simulink model "pv_model"  (R2024b)
settings: Solver=VariableStepAuto  StartTime=0.0  StopTime=1.5  RelTol=1e-3
libraries: simulink x1
settings Model: Creator=vasudha  LastModifiedBy=vasudha
settings DebuggingCC: AlgebraicLoopMsg=none

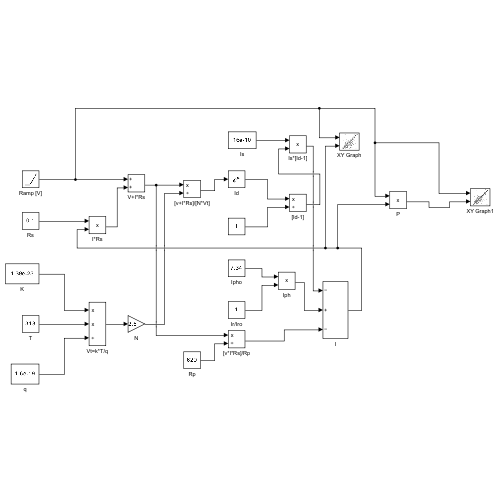
[thumbnail: Simulink's stored preview of the top-level diagram]
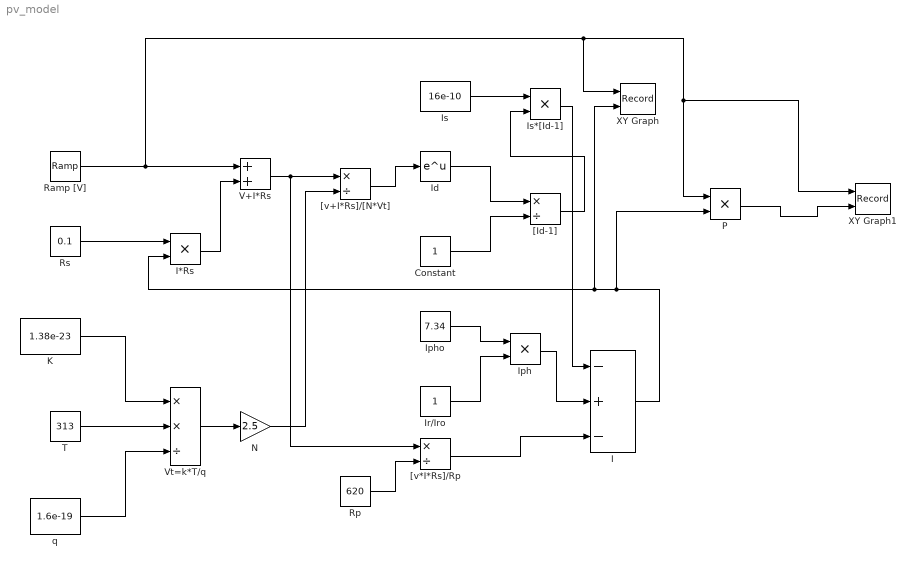
== system pv_model ==
  Constant : Constant
  I : Sum  Inputs=-+-
  I*Rs : Product
  Id : Math
  Iph : Product
  Ipho : Constant  Value=7.34
  Ir/Iro : Constant
  Is : Constant  Value=16e-10
  Is*[Id-1] : Product
  K : Constant  Value=1.38e-23
  N : Gain  Gain=2.5
  P : Product
  Ramp [V] : simulink/Sources/Ramp  slope=1  start=0  InitialOutput=0
  Rp : Constant  Value=620
  Rs : Constant  Value=0.1
  T : Constant  Value=313
  V+I*Rs : Sum
  Vt=k*T/q : Product  Inputs=**/
  XY Graph : Record  FileSettingsInternal="{\"entries\":[{\"content\":{\"excelSettings\":{\"content\":{},\"type\":\"Streamout.ExcelSettings\"}},\"type\":\"Streamout.FileSettingStorage\",\"uuid\":\"\"}],\"packageUris\":[\"http:\\/\\/schema.mathworks.com\\/mf0\\/streamout_blocks\\/R2020a\"],\"version\":\"1.0\"}"  Layout=[1 1]  SignalsInternal="{\"entries\":[{\"content\":{\"signals\":[{\"content\":{\"blockPath\":[],\"dimensions\":[1],\"domain\":\"\",\"lineColor\":\"#a2142f\",\"plots\":[ 1 ],\"port\":1,\"sid\":[\"\"],\"signalID\":1,\"signalName\":\"Ramp [V]\"},\"type\":\"RecordBlkView.Signal\",\"uuid\":\"\"},{\"content\":{\"blockPath\":[],\"dimensions\":[1],\"domain\":\"\",\"lineColor\":\"#139fff\",\"plots\":[ 1 ],\"port\":2,\"sid\":[\"\"],\"signalID\":2,\"signalName\":\"I\"},\"type\":\"RecordBlkView.Signal\",\"uuid\":\"\"}]},\"type\":\"RecordBlkView.InputSignals\",\"uuid\":\"\"}],\"packageUris\":[\"http:\\/\\/schema.mathworks.com\\/mf0\\/streamout_blocks\\/R2020a\"],\"version\":\"1.0\"}"  VisualizationBindings="{\"xyplotplugin\":{\"info\":[{\"series\":[{\"bindingParametersList\":[{\"parameter\":\"X-Axis\",\"signalID\":1,\"signalName\":\"Ramp [V]\"},{\"parameter\":\"Y-Axis\",\"signalID\":2,\"signalName\":\"I\"}],\"seriesID\":0}],\"subplotID\":1}]}}"  CompatibilityTag=XY
  XY Graph1 : Record  FileSettingsInternal="{\"entries\":[{\"content\":{\"excelSettings\":{\"content\":{},\"type\":\"Streamout.ExcelSettings\"}},\"type\":\"Streamout.FileSettingStorage\",\"uuid\":\"\"}],\"packageUris\":[\"http:\\/\\/schema.mathworks.com\\/mf0\\/streamout_blocks\\/R2020a\"],\"version\":\"1.0\"}"  Layout=[1 1]  SignalsInternal="{\"entries\":[{\"content\":{\"signals\":[{\"content\":{\"blockPath\":[],\"dimensions\":[1],\"domain\":\"\",\"lineColor\":\"#a2142f\",\"plots\":[ 1 ],\"port\":1,\"sid\":[\"\"],\"signalID\":1,\"signalName\":\"Ramp [V]\"},\"type\":\"RecordBlkView.Signal\",\"uuid\":\"\"},{\"content\":{\"blockPath\":[],\"dimensions\":[1],\"domain\":\"\",\"lineColor\":\"#139fff\",\"plots\":[ 1 ],\"port\":2,\"sid\":[\"\"],\"signalID\":2,\"signalName\":\"P\"},\"type\":\"RecordBlkView.Signal\",\"uuid\":\"\"}]},\"type\":\"RecordBlkView.InputSignals\",\"uuid\":\"\"}],\"packageUris\":[\"http:\\/\\/schema.mathworks.com\\/mf0\\/streamout_blocks\\/R2020a\"],\"version\":\"1.0\"}"  VisualizationBindings="{\"xyplotplugin\":{\"info\":[{\"series\":[{\"bindingParametersList\":[{\"parameter\":\"X-Axis\",\"signalID\":1,\"signalName\":\"Ramp [V]\"},{\"parameter\":\"Y-Axis\",\"signalID\":2,\"signalName\":\"P\"}],\"seriesID\":0}],\"subplotID\":1}]}}"  CompatibilityTag=XY
  "[Id-1]" : Product  Inputs=*/
  "[v*I*Rs]/Rp" : Product  Inputs=*/
  "[v+I*Rs]/[N*Vt]" : Product  Inputs=*/
  q : Constant  Value=1.6e-19
  wires:
  Rs/1 -> I*Rs/1
  K/1 -> Vt=k*T/q/1
  T/1 -> Vt=k*T/q/2
  q/1 -> Vt=k*T/q/3
  I*Rs/1 -> V+I*Rs/2
  V+I*Rs/1 -> "[v*I*Rs]/Rp"/1, "[v+I*Rs]/[N*Vt]"/1
  Vt=k*T/q/1 -> N/1
  N/1 -> "[v+I*Rs]/[N*Vt]"/2
  Rp/1 -> "[v*I*Rs]/Rp"/2
  "[v+I*Rs]/[N*Vt]"/1 -> Id/1
  Id/1 -> "[Id-1]"/1
  Constant/1 -> "[Id-1]"/2
  Ipho/1 -> Iph/1
  Ir/Iro/1 -> Iph/2
  Is/1 -> Is*[Id-1]/1
  "[Id-1]"/1 -> Is*[Id-1]/2
  Is*[Id-1]/1 -> I/1
  Iph/1 -> I/2
  "[v*I*Rs]/Rp"/1 -> I/3
  I/1 -> P/2, XY Graph/2, I*Rs/2
  P/1 -> XY Graph1/2
  Ramp [V]/1 -> XY Graph/1, XY Graph1/1, P/1, V+I*Rs/1
